simulink model "ep6_1_1"  (R2018a)
settings: Solver=VariableStepAuto  StartTime=0.0  StopTime=10.0  RelTol=1e-3
settings Model: Creator=zheny  LastModifiedBy=zheny

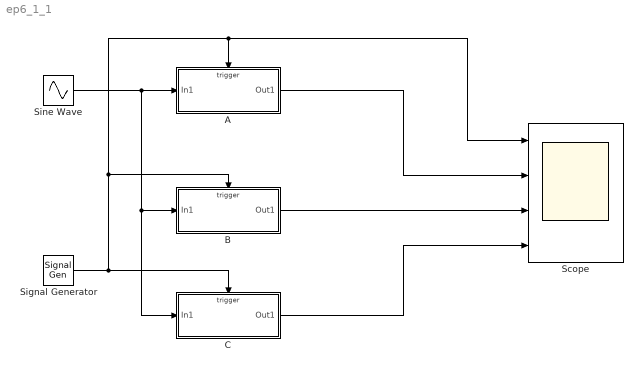
== system ep6_1_1 ==
  A : Subsystem  TreatAsAtomicUnit=on
  B : Subsystem  TreatAsAtomicUnit=on
  C : Subsystem  TreatAsAtomicUnit=on
  Scope : Scope  NumInputPorts=4
  Signal Generator : SignalGenerator  WaveForm=square
  Sine Wave : Sin  Frequency=8  SampleTime=0
  wires:
  B/1(Out1) -> Scope/3
  C/1(Out1) -> Scope/4
  Signal Generator/1 -> A/Trigger, Scope/1, B/Trigger, C/Trigger
  A/1(Out1) -> Scope/2
  Sine Wave/1 -> B/1(In1), C/1(In1), A/1(In1)

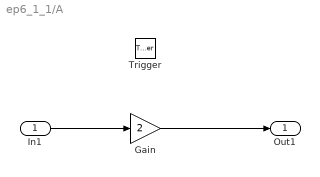
== system ep6_1_1/A ==
  In1 : Inport
  Trigger : TriggerPort  VariantControl=Variant
  Gain : Gain  Gain=2
  Out1 : Outport
  wires:
  In1/1 -> Gain/1
  Gain/1 -> Out1/1

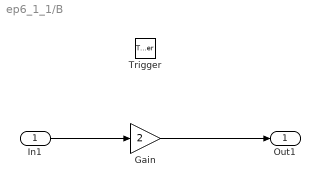
== system ep6_1_1/B ==
  In1 : Inport
  Trigger : TriggerPort  TriggerType=falling  VariantControl=Variant
  Gain : Gain  Gain=2
  Out1 : Outport
  wires:
  In1/1 -> Gain/1
  Gain/1 -> Out1/1

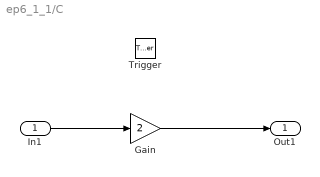
== system ep6_1_1/C ==
  In1 : Inport
  Trigger : TriggerPort  TriggerType=either  VariantControl=Variant
  Gain : Gain  Gain=2
  Out1 : Outport
  wires:
  In1/1 -> Gain/1
  Gain/1 -> Out1/1
